simulink model "BoundingBoxArea"  (R2016a)
settings: Solver=VariableStepAuto  StartTime=0.0  StopTime=inf  RelTol=1e-3
undefined symbols (not defined in the file): none, Rec, SDTV, videoinput
libraries: visionsinks x3, visionconversions x2, imaqlib x1
settings Model: Creator=YASARA  LastModifiedBy=YASARA

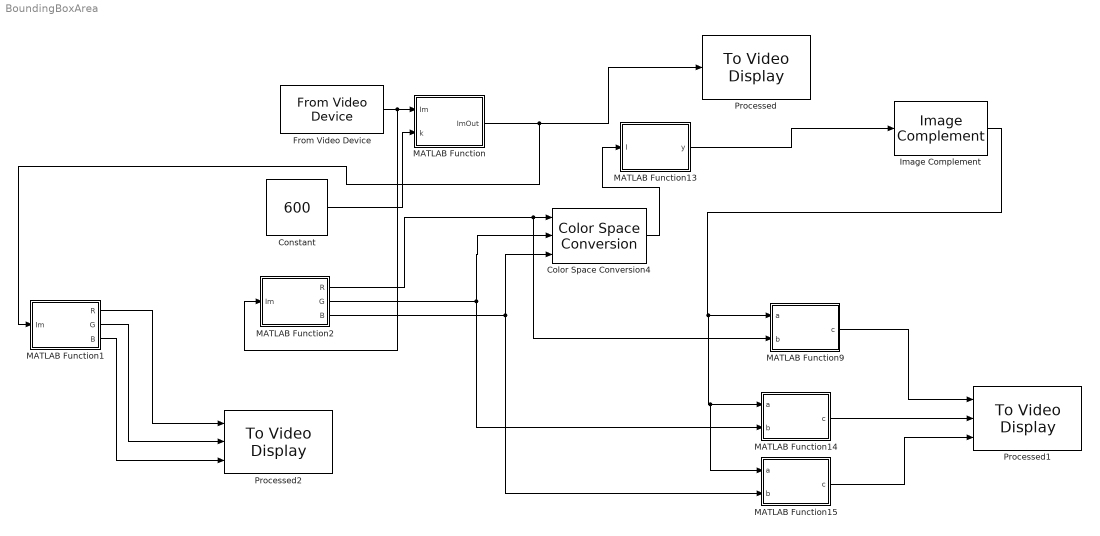
== system BoundingBoxArea ==
  Color Space Conversion4 : visionconversions/Color Space  Conversion  conversion=Obsolete  conversionActive=R'G'B' to intensity  wp_str=D65  rec=Rec. 601 (SDTV)  sys=1125/60/2:1  imagePorts=Separate color signals
  Constant : Constant  Value=600  OutDataTypeStr=uint32  SampleTime=100000
  From Video Device : imaqlib/From Video Device  DeviceMenu=winvideo 2 (USB Video Device)  Device=winvideo 2 (USB Video Device)  ObjConstructor=videoinput('winvideo', 2)  VideoFormatMenu=YUY2_160x120  VideoFormat=YUY2_160x120  VideoSource=input1  ROIPosition=[0 0 120 160]  EnableHWTrigger=off  TriggerConfiguration=none/none  SampleTime=1/30  OutputPortsMode=One multidimensional signal  DataType=double  CanDoHWTrigger=no  ReturnedColorSpace=rgb  BlockHandle=44.0042  ROIWidth=160  ROIHeight=120  ROIColumn=0  ROIRow=0  EngXMLPath=C:\Program Files\MATLAB\R2016a\toolbox\imaq\imaq\private  DevXMLPath=C:\MATLAB\SupportPackages\R2016a\toolbox\imaq\supportpackages\genericvideo\adaptor\win64  EngLibPath=C:\Program Files\MATLAB\R2016a\toolbox\imaq\imaqblks\imaqmex\win64  ColorSpace=rgb  BayerSensorAlignment=grbg
  Image Complement : visionconversions/Image Complement
  MATLAB Function : MATLAB Function  TreatAsAtomicUnit=on
  MATLAB Function1 : MATLAB Function  TreatAsAtomicUnit=on
  MATLAB Function13 : MATLAB Function  TreatAsAtomicUnit=on
  MATLAB Function14 : MATLAB Function  TreatAsAtomicUnit=on
  MATLAB Function15 : MATLAB Function  TreatAsAtomicUnit=on
  MATLAB Function2 : MATLAB Function  TreatAsAtomicUnit=on
  MATLAB Function9 : MATLAB Function  TreatAsAtomicUnit=on
  Processed : visionsinks/To Video Display  windowSizeMode=Normal  openAtMdlStart=on  fullScreen=off  videoWindowX=784  videoWindowY=165  saveWindowSize=off  videoWindowWidth=512  videoWindowHeight=384  inputColorFormat=RGB  inputType=Obsolete  imagePorts=One multidimensional signal  OutputDevice=On-screen video monitor  dataOrg=Column-major  isWindowOpen=off
  Processed1 : visionsinks/To Video Display  windowSizeMode=Normal  openAtMdlStart=on  fullScreen=off  videoWindowX=611  videoWindowY=290  saveWindowSize=off  videoWindowWidth=512  videoWindowHeight=384  inputColorFormat=RGB  inputType=Obsolete  imagePorts=Separate color signals  OutputDevice=On-screen video monitor  dataOrg=Column-major  isWindowOpen=off
  Processed2 : visionsinks/To Video Display  windowSizeMode=Normal  openAtMdlStart=on  fullScreen=off  videoWindowX=784  videoWindowY=165  saveWindowSize=off  videoWindowWidth=512  videoWindowHeight=384  inputColorFormat=RGB  inputType=Obsolete  imagePorts=Separate color signals  OutputDevice=On-screen video monitor  dataOrg=Column-major  isWindowOpen=off
  wires:
  From Video Device/1 -> MATLAB Function2/1(Im), MATLAB Function/1(Im)
  MATLAB Function/1(ImOut) -> MATLAB Function1/1(Im), Processed/1
  Constant/1 -> MATLAB Function/2(k)
  Color Space Conversion4/1 -> MATLAB Function13/1(I)
  MATLAB Function9/1(c) -> Processed1/1
  MATLAB Function14/1(c) -> Processed1/2
  MATLAB Function15/1(c) -> Processed1/3
  MATLAB Function2/1(R) -> MATLAB Function9/2(b), Color Space Conversion4/1
  MATLAB Function2/2(G) -> MATLAB Function14/2(b), Color Space Conversion4/2
  MATLAB Function2/3(B) -> MATLAB Function15/2(b), Color Space Conversion4/3
  MATLAB Function13/1(y) -> Image Complement/1
  Image Complement/1 -> MATLAB Function15/1(a), MATLAB Function14/1(a), MATLAB Function9/1(a)
  MATLAB Function1/1(R) -> Processed2/1
  MATLAB Function1/2(G) -> Processed2/2
  MATLAB Function1/3(B) -> Processed2/3

== matlab function BoundingBoxArea/MATLAB Function2 ==
  data: Im input; R output; G output; B output
function [R,G,B] = fcn(Im)
%#codegen
R=Im(:,:,1);
G=Im(:,:,2);
B=Im(:,:,3);

== matlab function BoundingBoxArea/MATLAB Function ==
  data: Im input; ImOut output; k input
function ImOut = fcn(Im,k)
I=rgb2gray(Im);
coder.extrinsic('graythresh');
coder.extrinsic('im2bw');
level = graythresh(I);
BW = im2bw(I,level);
L=double(I);
coder.extrinsic('bwlabeln');
NUM=1;
BW2=imcomplement(BW);
[L, NUM] = bwlabeln(BW2);
area=1;
n=1;
R1=Im(:,:,1);
R2=Im(:,:,2);
R3=Im(:,:,3);
AA=1;

for n=1:NUM
    [r, c] = find(L==n);
        AA=((max(r)-min(r))*(max(c)-min(c)));
        if AA<k
           R1(L==n)=0; 
           R2(L==n)=0;            
           R3(L==n)=255;
        end
end
II=Im;
II=cat(3,R1,R2,R3);
ImOut=II;

== matlab function BoundingBoxArea/MATLAB Function14 ==
  data: a input; b input; c output
function c = fcn(a,b)
%#codegen
c=a.*b;
return

== matlab function BoundingBoxArea/MATLAB Function1 ==
  data: Im input; R output; G output; B output
function [R,G,B] = fcn(Im)

R=double(Im(:,:,1));
G=double(Im(:,:,2));
B=double(Im(:,:,3));

== matlab function BoundingBoxArea/MATLAB Function13 ==
  data: I input; y output
function y = fcn(I)
%#codegen
y=I;
 coder.extrinsic('graythresh');
level = graythresh(I);
BW = double(im2bw(I,level));
y = BW;

== matlab function BoundingBoxArea/MATLAB Function15 ==
  data: a input; b input; c output
function c = fcn(a,b)
%#codegen
c=a.*b;
return

== matlab function BoundingBoxArea/MATLAB Function9 ==
  data: a input; b input; c output
function c = fcn(a,b)
%#codegen
c=a.*b;
return
